simulink model "Commande_2020"  (R2020b)
settings: Solver=FixedStepAuto  StartTime=0.0  StopTime=0.3  FixedStep=1e-6  RelTol=1e-3
libraries: powerlib x37, powerlib_meascontrol x9, spsFuelCellStackLib x4, fuzblock x3, powerlib_extras x2, simulink x1
settings Model: Creator=Abdelhak_Samir  LastModifiedBy=Abdelhak_Samir
settings SolverCC: ZeroCrossAlgorithm=Adaptive
settings DebuggingCC: IgnoredZcDiagnostic=none  UnconnectedInputMsg=none  UnconnectedOutputMsg=none  UnconnectedLineMsg=none
settings ModelReferenceCC: EnableRefExpFcnMdlSchedulingChecks=off
settings RTWCC: GPUComputeCapability=5.0

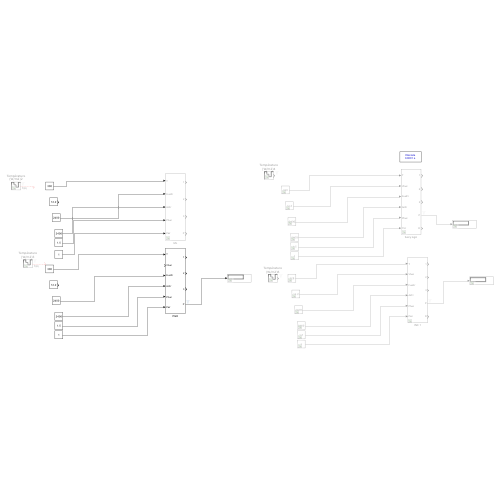
[thumbnail: Simulink's stored preview of the top-level diagram]
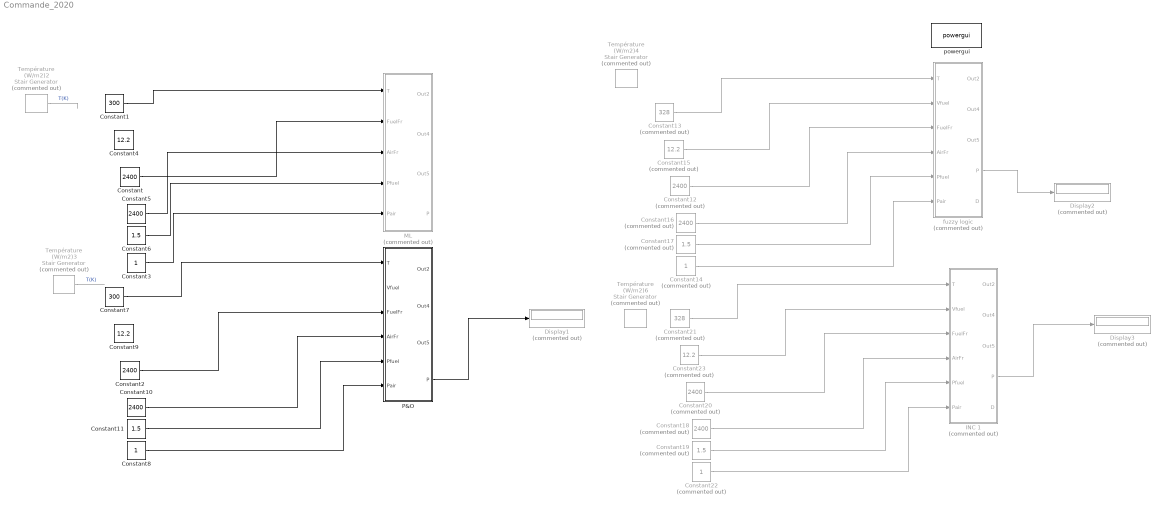
== system Commande_2020 ==
  Constant{,2,5,10} (4 alike) : Constant  Value=2400
  Constant1 : Constant  Value=300
  Constant11 : Constant  Value=1.5
  Constant{12,16,18,20} (4 alike) : Constant  Commented=on  Value=2400
  Constant13 : Constant  Commented=on  Value=328
  Constant14 : Constant  Commented=on
  Constant15 : Constant  Commented=on  Value=12.2
  Constant17 : Constant  Commented=on  Value=1.5
  Constant19 : Constant  Commented=on  Value=1.5
  Constant21 : Constant  Commented=on  Value=328
  Constant22 : Constant  Commented=on
  Constant23 : Constant  Commented=on  Value=12.2
  Constant3 : Constant
  Constant4 : Constant  Value=12.2
  Constant6 : Constant  Value=1.5
  Constant7 : Constant  Value=300
  Constant8 : Constant
  Constant9 : Constant  Value=12.2
  Display1 : Display  Commented=on
  Display2 : Display  Commented=on
  Display3 : Display  Commented=on
  INC 1 : Subsystem  Commented=on
  ML : Subsystem  Commented=on
  P&O : Subsystem
  Température (W/m2){2..4,6} (4 alike) : powerlib_meascontrol/Pulse & Signal Generators/Stair Generator  Commented=on  t=[0, 0.2 , 0.4 , 0.6, 0.8,1]  e=[300,330,320,310,330,330]  Ts=0.00001
  fuzzy logic : Subsystem  Commented=on
  powergui : powerlib/powergui  Priority=1  SimulationMode=Discrete  SampleTime=1e-4  frequency=60  Iterations=50  frequencyindice=0  Pbase=100e6  ErrMax=1e-4  UnitsV=kV  UnitsW=MW  buscounter=0  FunctionMessages=off  echomessages=off  EnableUseOfTLC=off  CurrentSourceSwitches=off  DisableSnubberDevices=off  DisableRonSwitches=off  DisableVfSwitches=off  DisplayEquations=off  AutomaticDiscreteSolvers=off  SolverType=Tustin/Backward Euler (TBE)  Interpol=off  ExternalGateDelay=off  methode=off  Ts=100  x0status=blocks  SPID=on  SwTol=0  HookPort=off  NonlinearTolerance=1e-4  nMaxIteration=100  ContinueOnMaxIteration=off  RestoreLinks=warning  ResistiveCurrentMeasurement=off  Frange=[0:2:500]  Ylog=off  Xlog=on  ShowGrid=off  save=off  variable=ZData  structure=0  ZoomFFT=off  StartTime=0.0  cycles=1  DisplayStyle=1  fundamental=60  FreqAxis=off  MaxFrequency=1000  frequencyindicesteady=1  RmsSteady=1  display=off
  wires:
  Constant8/1 -> P&O/6(Pair)
  Constant10/1 -> P&O/4(AirFr)
  P&O/4(P) -> Display1/1
  Constant11/1 -> P&O/5(Pfuel)
  Constant14/1 -> fuzzy logic/6(Pair)
  Constant12/1 -> fuzzy logic/3(FuelFr)
  Constant15/1 -> fuzzy logic/2(Vfuel)
  Constant16/1 -> fuzzy logic/4(AirFr)
  fuzzy logic/4(P) -> Display2/1
  Constant17/1 -> fuzzy logic/5(Pfuel)
  INC 1/4(P) -> Display3/1
  Constant18/1 -> INC 1/4(AirFr)
  Constant20/1 -> INC 1/3(FuelFr)
  Constant22/1 -> INC 1/6(Pair)
  Constant23/1 -> INC 1/2(Vfuel)
  Constant19/1 -> INC 1/5(Pfuel)
  Constant1/1 -> ML/1(T)
  Constant7/1 -> P&O/1(T)
  Constant13/1 -> fuzzy logic/1(T)
  Constant21/1 -> INC 1/1(T)
  Constant3/1 -> ML/5(Pair)
  Constant6/1 -> ML/4(Pfuel)
  Constant5/1 -> ML/3(AirFr)
  Constant/1 -> ML/2(FuelFr)
  Température (W/m2)2/1 -> ?  "T(K)"
  Température (W/m2)3/1 -> ?  "T(K)"
  Constant2/1 -> P&O/3(FuelFr)

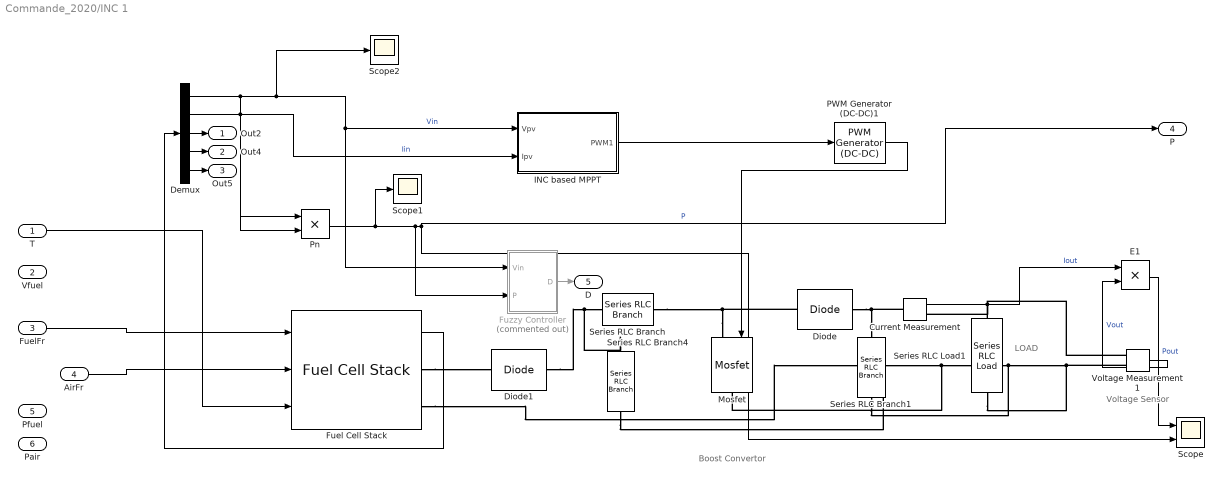
== system Commande_2020/INC 1 ==
  note: LOAD
  note: Boost Convertor
  note: Voltage Sensor
  T : Inport
  Vfuel : Inport  Port=2
  FuelFr : Inport  Port=3
  AirFr : Inport  Port=4
  Pfuel : Inport  Port=5
  Pair : Inport  Port=6
  Current Measurement : powerlib/Measurements/Current Measurement  PhasorSimulation=off  OutputType=Complex  PSBequivalent=0
  Demux : Demux  Outputs=5
  Diode : powerlib/Power Electronics/Diode  Ron=0.001  Lon=0  Vf=0.7  IC=0  UseSnubber=0  Rs=500  Cs=250e-9  Measurements=off
  Diode1 : powerlib/Power Electronics/Diode  Ron=0.001  Lon=0  Vf=0.7  IC=0  UseSnubber=0  Rs=500  Cs=250e-9  Measurements=off
  E1 : Product  Inputs=**
  Fuel Cell Stack : spsFuelCellStackLib/Fuel Cell Stack  PresetModel=No (User-Defined)  FcType=0  Detailed=Detailed  Eoc=[42,35]  NomVI=[52,24.23]  EndVI=[100,20]  Nc=1  n=46  TOp=55  AirFr=2400  SuppPress=[1.5,1]  Comp=[99.95,21,1]  SignX=off  SignY=off  FlowRateH2=on  FlowRateAir=on  SystemTemp=on  SystemPH2=off  SystemPAir=off  FCDyn=off  FC_tau=1  Peak_O2=80  V_Under=10
  Fuzzy Controller : Subsystem  Commented=on
  INC based MPPT : Subsystem
  Mosfet : powerlib/Power Electronics/Mosfet  Ron=0.1  Lon=0  Rd=0.01  Vfd=0.7  IC=0  Rs=1e5  Cs=10^-9  Measurements=off
  PWM Generator (DC-DC)1 : powerlib_meascontrol/Pulse & Signal Generators/PWM Generator (DC-DC)  Fsw=10000  Ts=0
  Pn : Product
  Scope : Scope  NumInputPorts=2
  Scope1 : Scope
  Scope2 : Scope
  Series RLC Branch : powerlib/Elements/Series RLC Branch  LConnTagsString=__new0  RConnTagsString=__new0  BranchType=L  Resistance=1  Inductance=1e-4  SetiL0=off  InitialCurrent=0  Capacitance=1e-6  Setx0=off  InitialVoltage=0  Measurements=None
  Series RLC Branch1 : powerlib/Elements/Series RLC Branch  LConnTagsString=__new0  RConnTagsString=__new0  BranchType=C  Resistance=1  Inductance=1e-4  SetiL0=off  InitialCurrent=0  Capacitance=4700e-6  Setx0=off  InitialVoltage=0  Measurements=None
  Series RLC Branch4 : powerlib/Elements/Series RLC Branch  LConnTagsString=__new0  RConnTagsString=__new0  BranchType=C  Resistance=1  Inductance=1e-4  SetiL0=off  InitialCurrent=0  Capacitance=4700e-5  Setx0=on  InitialVoltage=42  Measurements=None
  Series RLC Load1 : powerlib/Elements/Series RLC Load  LConnTagsString=a  RConnTagsString=__new0  NominalVoltage=50  NominalFrequency=500  ActivePower=33  InductivePower=0  CapacitivePower=0  Setx0=off  InitialVoltage=0  SetiL0=off  InitialCurrent=0  Measurements=None  LoadType=constant Z
  Voltage Measurement1 : powerlib/Measurements/Voltage Measurement  PhasorSimulation=off  OutputType=Complex  PSBequivalent=0
  Out2 : Outport
  Out4 : Outport  Port=2
  Out5 : Outport  Port=3
  P : Outport  Port=4
  D : Outport  Port=5
  wires:
  Current Measurement/1 -> E1/1  "Iout"
  Pn/1 -> P/1, Scope/2, Fuzzy Controller/2(P), Scope1/1  "P"
  PWM Generator (DC-DC)1/1 -> Mosfet/1
  Demux/1 -> Fuzzy Controller/1(Vin), INC based MPPT/1(Vpv), Scope2/1, Pn/1  "Vin"
  Fuzzy Controller/1(D) -> D/1
  Demux/5 -> Out5/1
  Demux/2 -> INC based MPPT/2(Ipv), Pn/2  "Iin"
  FuelFr/1 -> Fuel Cell Stack/1
  Fuel Cell Stack/1 -> Demux/1
  E1/1 -> Scope/1  "Pout"
  AirFr/1 -> Fuel Cell Stack/2
  Voltage Measurement1/1 -> E1/2  "Vout"
  INC based MPPT/1(PWM1) -> PWM Generator (DC-DC)1/1
  Demux/3 -> Out2/1
  Demux/4 -> Out4/1
  T/1 -> Fuel Cell Stack/3
  connections:
  Series RLC Branch4/LConn1 -- Series RLC Branch/LConn1 -- Diode1/RConn1
  Series RLC Branch1/LConn1 -- Diode/RConn1 -- Current Measurement/LConn1
  Fuel Cell Stack/RConn1 -- Diode1/LConn1
  Mosfet/RConn1 -- Fuel Cell Stack/RConn2 -- Series RLC Branch4/RConn1 -- Voltage Measurement1/LConn2 -- Series RLC Load1/RConn1 -- Series RLC Branch1/RConn1
  Current Measurement/RConn1 -- Series RLC Load1/LConn1 -- Voltage Measurement1/LConn1
  Mosfet/LConn1 -- Diode/LConn1 -- Series RLC Branch/RConn1

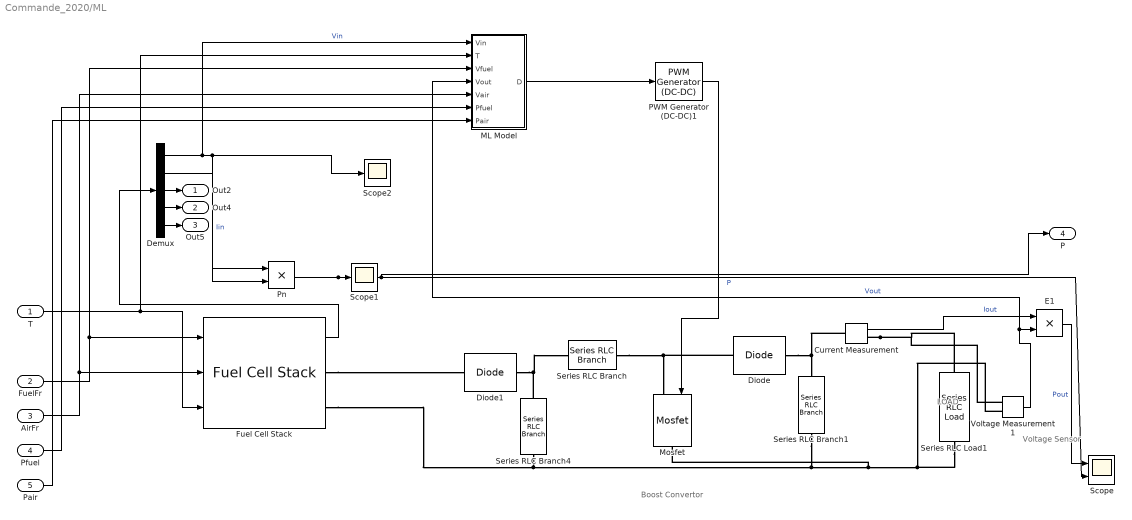
== system Commande_2020/ML ==
  note: LOAD
  note: Voltage Sensor
  note: Boost Convertor
  T : Inport
  FuelFr : Inport  Port=2
  AirFr : Inport  Port=3
  Pfuel : Inport  Port=4
  Pair : Inport  Port=5
  Current Measurement : powerlib/Measurements/Current Measurement  PhasorSimulation=off  OutputType=Complex  PSBequivalent=0
  Demux : Demux  Outputs=5
  Diode : powerlib/Power Electronics/Diode  Ron=0.001  Lon=0  Vf=0.7  IC=0  UseSnubber=0  Rs=500  Cs=250e-9  Measurements=off
  Diode1 : powerlib/Power Electronics/Diode  Ron=0.001  Lon=0  Vf=0.7  IC=0  UseSnubber=0  Rs=500  Cs=250e-9  Measurements=off
  E1 : Product  Inputs=**
  Fuel Cell Stack : spsFuelCellStackLib/Fuel Cell Stack  PresetModel=PEMFC - 1.26 kW - 24 Vdc  FcType=0  Detailed=Detailed  Eoc=[42,35]  NomVI=[52,24.23]  EndVI=[100,20]  Nc=42  n=46  TOp=55  AirFr=2400  SuppPress=[1.5,1]  Comp=[99.95,21,1]  SignX=off  SignY=off  FlowRateH2=on  FlowRateAir=on  SystemTemp=on  SystemPH2=off  SystemPAir=off  FCDyn=off  FC_tau=1  Peak_O2=80  V_Under=10
  ML Model : Subsystem
  Mosfet : powerlib/Power Electronics/Mosfet  Ron=0.1  Lon=0  Rd=0.01  Vfd=0.7  IC=0  Rs=1e5  Cs=10^-9  Measurements=off
  PWM Generator (DC-DC)1 : powerlib_meascontrol/Pulse & Signal Generators/PWM Generator (DC-DC)  Fsw=10000  Ts=0
  Pn : Product
  Scope : Scope  NumInputPorts=2
  Scope1 : Scope
  Scope2 : Scope
  Series RLC Branch : powerlib/Elements/Series RLC Branch  LConnTagsString=__new0  RConnTagsString=__new0  BranchType=L  Resistance=1  Inductance=1e-4  SetiL0=off  InitialCurrent=0  Capacitance=1e-6  Setx0=off  InitialVoltage=0  Measurements=None
  Series RLC Branch1 : powerlib/Elements/Series RLC Branch  LConnTagsString=__new0  RConnTagsString=__new0  BranchType=C  Resistance=1  Inductance=1e-4  SetiL0=off  InitialCurrent=0  Capacitance=4700e-6  Setx0=off  InitialVoltage=0  Measurements=None
  Series RLC Branch4 : powerlib/Elements/Series RLC Branch  LConnTagsString=__new0  RConnTagsString=__new0  BranchType=C  Resistance=1  Inductance=1e-4  SetiL0=off  InitialCurrent=0  Capacitance=4700e-5  Setx0=on  InitialVoltage=42  Measurements=None
  Series RLC Load1 : powerlib/Elements/Series RLC Load  LConnTagsString=a  RConnTagsString=__new0  NominalVoltage=50  NominalFrequency=500  ActivePower=33  InductivePower=0  CapacitivePower=0  Setx0=off  InitialVoltage=0  SetiL0=off  InitialCurrent=0  Measurements=None  LoadType=constant Z
  Voltage Measurement1 : powerlib/Measurements/Voltage Measurement  PhasorSimulation=off  OutputType=Complex  PSBequivalent=0
  Out2 : Outport
  Out4 : Outport  Port=2
  Out5 : Outport  Port=3
  P : Outport  Port=4
  wires:
  Pair/1 -> ML Model/7(Pair)
  FuelFr/1 -> Fuel Cell Stack/1, ML Model/3(Vfuel)
  T/1 -> Fuel Cell Stack/3, ML Model/2(T)
  Fuel Cell Stack/1 -> Demux/1
  Demux/3 -> Out2/1
  Demux/2 -> Pn/2  "Iin"
  Demux/5 -> Out5/1
  E1/1 -> Scope/1  "Pout"
  Pfuel/1 -> ML Model/6(Pfuel)
  Demux/4 -> Out4/1
  Current Measurement/1 -> E1/1  "Iout"
  AirFr/1 -> Fuel Cell Stack/2, ML Model/5(Vair)
  Voltage Measurement1/1 -> ML Model/4(Vout), E1/2  "Vout"
  Pn/1 -> P/1, Scope/2, Scope1/1  "P"
  Demux/1 -> ML Model/1(Vin), Scope2/1, Pn/1  "Vin"
  ML Model/1(D) -> PWM Generator (DC-DC)1/1
  PWM Generator (DC-DC)1/1 -> Mosfet/1
  connections:
  Diode1/RConn1 -- Series RLC Branch4/LConn1 -- Series RLC Branch/LConn1
  Current Measurement/LConn1 -- Series RLC Branch1/LConn1 -- Diode/RConn1
  Series RLC Branch4/RConn1 -- Fuel Cell Stack/RConn2 -- Series RLC Load1/RConn1 -- Voltage Measurement1/LConn2 -- Mosfet/RConn1 -- Series RLC Branch1/RConn1
  Current Measurement/RConn1 -- Series RLC Load1/LConn1 -- Voltage Measurement1/LConn1
  Series RLC Branch/RConn1 -- Diode/LConn1 -- Mosfet/LConn1
  Fuel Cell Stack/RConn1 -- Diode1/LConn1

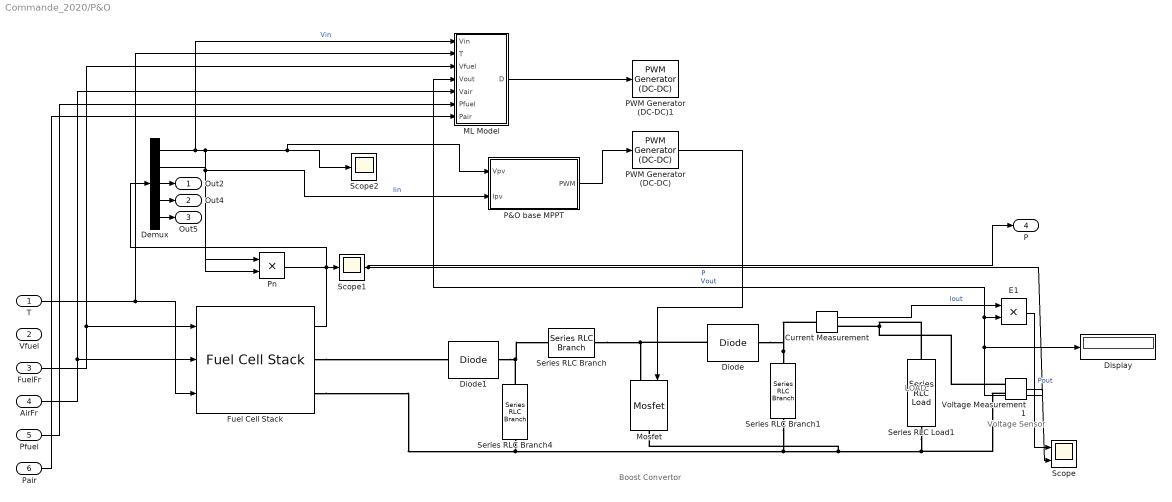
== system Commande_2020/P&O ==
  note: LOAD
  note: Boost Convertor
  note: Voltage Sensor
  T : Inport
  Vfuel : Inport  Port=2
  FuelFr : Inport  Port=3
  AirFr : Inport  Port=4
  Pfuel : Inport  Port=5
  Pair : Inport  Port=6
  Current Measurement : powerlib/Measurements/Current Measurement  PhasorSimulation=off  OutputType=Complex  PSBequivalent=0
  Demux : Demux  Outputs=5
  Diode : powerlib/Power Electronics/Diode  Ron=0.001  Lon=0  Vf=0.7  IC=0  UseSnubber=0  Rs=500  Cs=250e-9  Measurements=off
  Diode1 : powerlib/Power Electronics/Diode  Ron=0.001  Lon=0  Vf=0.7  IC=0  UseSnubber=0  Rs=500  Cs=250e-9  Measurements=off
  Display : Display
  E1 : Product  Inputs=**
  Fuel Cell Stack : spsFuelCellStackLib/Fuel Cell Stack  PresetModel=PEMFC - 1.26 kW - 24 Vdc  FcType=0  Detailed=Detailed  Eoc=[42,35]  NomVI=[52,24.23]  EndVI=[100,20]  Nc=42  n=46  TOp=55  AirFr=2400  SuppPress=[1.5,1]  Comp=[99.95,21,1]  SignX=off  SignY=off  FlowRateH2=on  FlowRateAir=on  SystemTemp=on  SystemPH2=off  SystemPAir=off  FCDyn=off  FC_tau=1  Peak_O2=80  V_Under=10
  ML Model : Subsystem
  Mosfet : powerlib/Power Electronics/Mosfet  Ron=0.1  Lon=0  Rd=0.01  Vfd=0.7  IC=0  Rs=1e5  Cs=10^-9  Measurements=off
  P&O base MPPT : Subsystem
  PWM Generator (DC-DC) : powerlib_meascontrol/Pulse & Signal Generators/PWM Generator (DC-DC)  Fsw=10000  Ts=1e-4
  PWM Generator (DC-DC)1 : powerlib_meascontrol/Pulse & Signal Generators/PWM Generator (DC-DC)  Fsw=10000  Ts=1e-4
  Pn : Product
  Scope : Scope  NumInputPorts=2
  Scope1 : Scope
  Scope2 : Scope
  Series RLC Branch : powerlib/Elements/Series RLC Branch  LConnTagsString=__new0  RConnTagsString=__new0  BranchType=L  Resistance=1  Inductance=1e-4  SetiL0=off  InitialCurrent=0  Capacitance=1e-6  Setx0=off  InitialVoltage=0  Measurements=None
  Series RLC Branch1 : powerlib/Elements/Series RLC Branch  LConnTagsString=__new0  RConnTagsString=__new0  BranchType=C  Resistance=1  Inductance=1e-4  SetiL0=off  InitialCurrent=0  Capacitance=4700e-6  Setx0=off  InitialVoltage=0  Measurements=None
  Series RLC Branch4 : powerlib/Elements/Series RLC Branch  LConnTagsString=__new0  RConnTagsString=__new0  BranchType=C  Resistance=1  Inductance=1e-4  SetiL0=off  InitialCurrent=0  Capacitance=4700e-5  Setx0=on  InitialVoltage=42  Measurements=None
  Series RLC Load1 : powerlib/Elements/Series RLC Load  LConnTagsString=a  RConnTagsString=__new0  NominalVoltage=50  NominalFrequency=500  ActivePower=33  InductivePower=0  CapacitivePower=0  Setx0=off  InitialVoltage=0  SetiL0=off  InitialCurrent=0  Measurements=None  LoadType=constant Z
  Voltage Measurement1 : powerlib/Measurements/Voltage Measurement  PhasorSimulation=off  OutputType=Complex  PSBequivalent=0
  Out2 : Outport
  Out4 : Outport  Port=2
  Out5 : Outport  Port=3
  P : Outport  Port=4
  wires:
  Current Measurement/1 -> E1/1  "Iout"
  Pn/1 -> P/1, Scope/2, Scope1/1  "P"
  Demux/1 -> ML Model/1(Vin), Scope2/1, P&O base MPPT/1(Vpv), Pn/1  "Vin"
  Demux/5 -> Out5/1
  Demux/2 -> P&O base MPPT/2(Ipv), Pn/2  "Iin"
  FuelFr/1 -> Fuel Cell Stack/1, ML Model/3(Vfuel)
  Fuel Cell Stack/1 -> Demux/1
  E1/1 -> Scope/1  "Pout"
  AirFr/1 -> Fuel Cell Stack/2, ML Model/5(Vair)
  Voltage Measurement1/1 -> Display/1, ML Model/4(Vout), E1/2  "Vout"
  Demux/3 -> Out2/1
  Demux/4 -> Out4/1
  T/1 -> ML Model/2(T), Fuel Cell Stack/3
  P&O base MPPT/1(PWM) -> PWM Generator (DC-DC)/1
  ML Model/1(D) -> PWM Generator (DC-DC)1/1
  Pfuel/1 -> ML Model/6(Pfuel)
  Pair/1 -> ML Model/7(Pair)
  PWM Generator (DC-DC)/1 -> Mosfet/1
  connections:
  Series RLC Branch4/LConn1 -- Series RLC Branch/LConn1 -- Diode1/RConn1
  Series RLC Branch1/LConn1 -- Diode/RConn1 -- Current Measurement/LConn1
  Fuel Cell Stack/RConn1 -- Diode1/LConn1
  Fuel Cell Stack/RConn2 -- Voltage Measurement1/LConn2 -- Series RLC Load1/RConn1 -- Mosfet/RConn1 -- Series RLC Branch1/RConn1 -- Series RLC Branch4/RConn1
  Series RLC Load1/LConn1 -- Voltage Measurement1/LConn1 -- Current Measurement/RConn1
  Diode/LConn1 -- Mosfet/LConn1 -- Series RLC Branch/RConn1

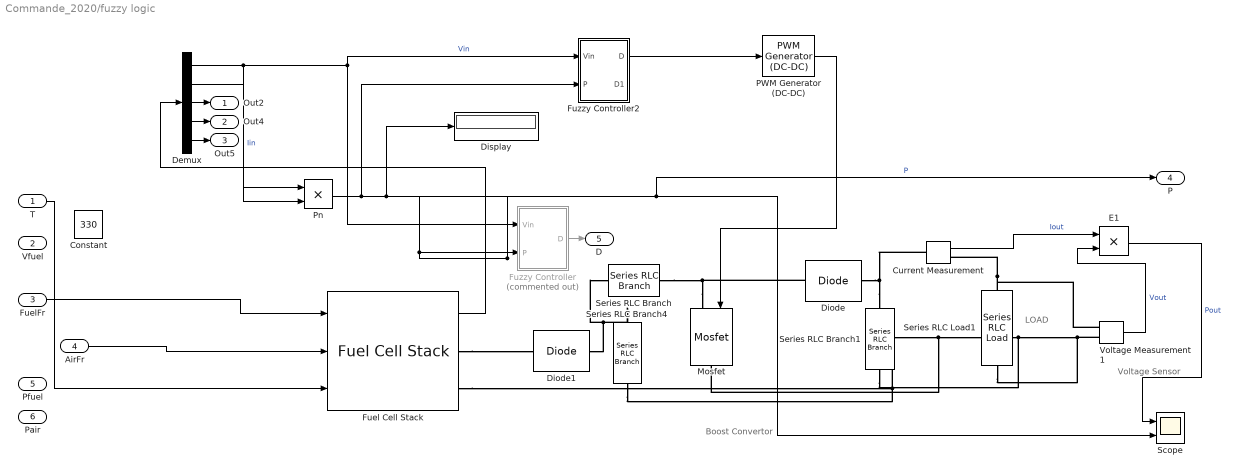
== system Commande_2020/fuzzy logic ==
  note: LOAD
  note: Boost Convertor
  note: Voltage Sensor
  T : Inport
  Vfuel : Inport  Port=2
  FuelFr : Inport  Port=3
  AirFr : Inport  Port=4
  Pfuel : Inport  Port=5
  Pair : Inport  Port=6
  Constant : Constant  Value=330
  Current Measurement : powerlib/Measurements/Current Measurement  PhasorSimulation=off  OutputType=Complex  PSBequivalent=0
  Demux : Demux  Outputs=5
  Diode : powerlib/Power Electronics/Diode  Ron=0.001  Lon=0  Vf=0.7  IC=0  UseSnubber=0  Rs=500  Cs=250e-9  Measurements=off
  Diode1 : powerlib/Power Electronics/Diode  Ron=0.001  Lon=0  Vf=0.7  IC=0  UseSnubber=0  Rs=500  Cs=250e-9  Measurements=off
  Display : Display
  E1 : Product  Inputs=**
  Fuel Cell Stack : spsFuelCellStackLib/Fuel Cell Stack  PresetModel=No (User-Defined)  FcType=0  Detailed=Detailed  Eoc=[42,35]  NomVI=[52,24.23]  EndVI=[100,20]  Nc=1  n=46  TOp=55  AirFr=2400  SuppPress=[1.5,1]  Comp=[99.95,21,1]  SignX=off  SignY=off  FlowRateH2=on  FlowRateAir=on  SystemTemp=on  SystemPH2=off  SystemPAir=off  FCDyn=off  FC_tau=1  Peak_O2=80  V_Under=10
  Fuzzy Controller : Subsystem  Commented=on
  Fuzzy Controller2 : Subsystem
  Mosfet : powerlib/Power Electronics/Mosfet  Ron=0.1  Lon=0  Rd=0.01  Vfd=0.7  IC=0  Rs=1e5  Cs=10^-9  Measurements=off
  PWM Generator (DC-DC) : powerlib_meascontrol/Pulse & Signal Generators/PWM Generator (DC-DC)  Fsw=10000  Ts=0
  Pn : Product
  Scope : Scope  NumInputPorts=2
  Series RLC Branch : powerlib/Elements/Series RLC Branch  LConnTagsString=__new0  RConnTagsString=__new0  BranchType=L  Resistance=1  Inductance=1e-4  SetiL0=off  InitialCurrent=0  Capacitance=1e-6  Setx0=off  InitialVoltage=0  Measurements=None
  Series RLC Branch1 : powerlib/Elements/Series RLC Branch  LConnTagsString=__new0  RConnTagsString=__new0  BranchType=C  Resistance=1  Inductance=1e-4  SetiL0=off  InitialCurrent=0  Capacitance=4700e-6  Setx0=off  InitialVoltage=0  Measurements=None
  Series RLC Branch4 : powerlib/Elements/Series RLC Branch  LConnTagsString=__new0  RConnTagsString=__new0  BranchType=C  Resistance=1  Inductance=1e-4  SetiL0=off  InitialCurrent=0  Capacitance=4700e-5  Setx0=on  InitialVoltage=42  Measurements=None
  Series RLC Load1 : powerlib/Elements/Series RLC Load  LConnTagsString=a  RConnTagsString=__new0  NominalVoltage=50  NominalFrequency=500  ActivePower=33  InductivePower=0  CapacitivePower=0  Setx0=off  InitialVoltage=0  SetiL0=off  InitialCurrent=0  Measurements=None  LoadType=constant Z
  Voltage Measurement1 : powerlib/Measurements/Voltage Measurement  PhasorSimulation=off  OutputType=Complex  PSBequivalent=0
  Out2 : Outport
  Out4 : Outport  Port=2
  Out5 : Outport  Port=3
  P : Outport  Port=4
  D : Outport  Port=5
  wires:
  Current Measurement/1 -> E1/1  "Iout"
  Pn/1 -> Fuzzy Controller2/2(P), Display/1, P/1, Scope/2, Fuzzy Controller/2(P)  "P"
  Demux/1 -> Fuzzy Controller2/1(Vin), Fuzzy Controller/1(Vin), Pn/1  "Vin"
  Fuzzy Controller/1(D) -> D/1
  Demux/5 -> Out5/1
  Demux/2 -> Pn/2  "Iin"
  Fuel Cell Stack/1 -> Demux/1
  E1/1 -> Scope/1  "Pout"
  Voltage Measurement1/1 -> E1/2  "Vout"
  PWM Generator (DC-DC)/1 -> Mosfet/1
  Demux/3 -> Out2/1
  Demux/4 -> Out4/1
  Fuzzy Controller2/1(D) -> PWM Generator (DC-DC)/1
  AirFr/1 -> Fuel Cell Stack/2
  FuelFr/1 -> Fuel Cell Stack/1
  T/1 -> Fuel Cell Stack/3
  connections:
  Series RLC Branch4/LConn1 -- Series RLC Branch/LConn1 -- Diode1/RConn1
  Series RLC Branch1/LConn1 -- Diode/RConn1 -- Current Measurement/LConn1
  Fuel Cell Stack/RConn1 -- Diode1/LConn1
  Mosfet/RConn1 -- Fuel Cell Stack/RConn2 -- Series RLC Branch4/RConn1 -- Series RLC Load1/RConn1 -- Voltage Measurement1/LConn2 -- Series RLC Branch1/RConn1
  Current Measurement/RConn1 -- Voltage Measurement1/LConn1 -- Series RLC Load1/LConn1
  Mosfet/LConn1 -- Diode/LConn1 -- Series RLC Branch/RConn1

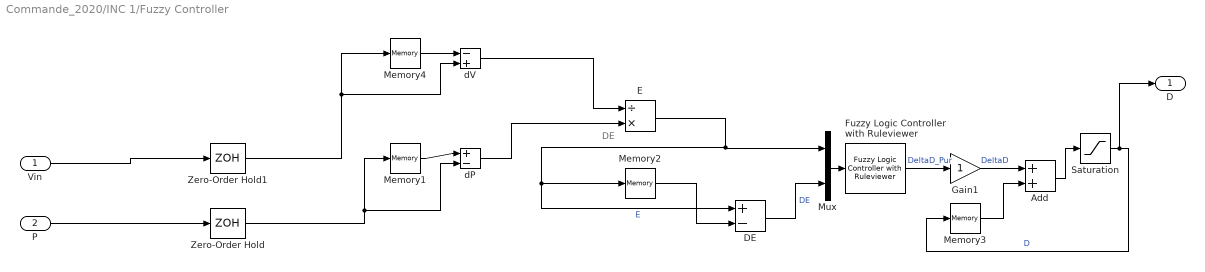
== system Commande_2020/INC 1/Fuzzy Controller ==
  note: DE
  Vin : Inport
  P : Inport  Port=2
  Add : Sum
  DE : Sum  Inputs=+-
  E : Product  Inputs=/*
  Fuzzy Logic Controller with Ruleviewer : fuzblock/Fuzzy Logic  Controller  with Ruleviewer  fismatrix=twnty_five_rules_2  Ts=0.1
  Gain1 : Gain
  Memory1 : Memory  InheritSampleTime=on
  Memory2 : Memory  InheritSampleTime=on
  Memory3 : Memory
  Memory4 : Memory  InheritSampleTime=on
  Mux : Mux  Inputs=2
  Saturation : Saturate  UpperLimit=0.9  LowerLimit=0.1
  Zero-Order Hold : ZeroOrderHold  SampleTime=-1
  Zero-Order Hold1 : ZeroOrderHold  SampleTime=-1
  dP : Sum  Inputs=|+-
  dV : Sum  Inputs=-+
  D : Outport
  wires:
  DE/1 -> Mux/2  "DE"
  Fuzzy Logic Controller with Ruleviewer/1 -> Gain1/1  "DeltaD_Pur"
  Zero-Order Hold/1 -> dP/2, Memory1/1
  dV/1 -> E/1
  dP/1 -> E/2
  E/1 -> DE/1, Memory2/1, Mux/1  "E"
  Mux/1 -> Fuzzy Logic Controller with Ruleviewer/1
  Memory4/1 -> dV/1
  Memory1/1 -> dP/1
  Zero-Order Hold1/1 -> Memory4/1, dV/2
  Gain1/1 -> Add/1  "DeltaD"
  Memory3/1 -> Add/2
  Saturation/1 -> D/1, Memory3/1  "D"
  Memory2/1 -> DE/2
  Add/1 -> Saturation/1
  Vin/1 -> Zero-Order Hold1/1
  P/1 -> Zero-Order Hold/1

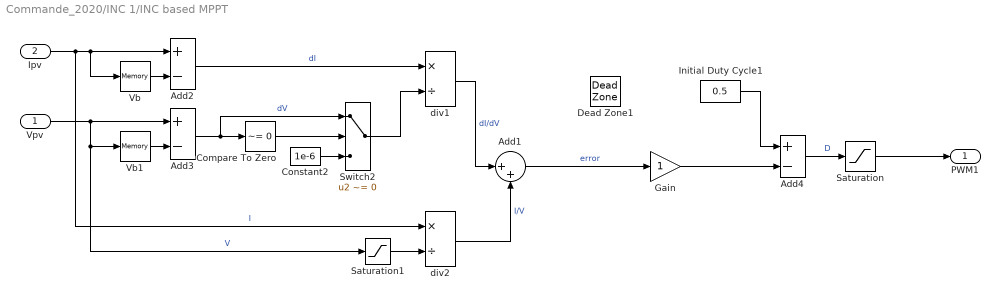
== system Commande_2020/INC 1/INC based MPPT ==
  Vpv : Inport
  Ipv : Inport  Port=2
  Add1 : Sum  Inputs=|++
  Add2 : Sum  Inputs=+-
  Add3 : Sum  Inputs=+-
  Add4 : Sum  Inputs=+-
  Compare To Zero : simulink/Logic and Bit Operations/Compare To Zero  relop=~=  OutDataTypeStr=uint8
  Constant2 : Constant  Value=1e-6
  Dead Zone1 : DeadZone  LowerValue=-0.02  UpperValue=+0.02  SaturateOnIntegerOverflow=on
  Gain : Gain
  Initial Duty Cycle1 : Constant  Value=0.5
  Saturation : Saturate  UpperLimit=0.9  LowerLimit=0.1
  Saturation1 : Saturate  UpperLimit=inf  LowerLimit=eps
  Switch2 : Switch  Criteria=u2 ~= 0
  Vb : Memory  InheritSampleTime=on  LinearizeAsDelay=on
  Vb1 : Memory  InheritSampleTime=on  LinearizeAsDelay=on
  div1 : Product  Inputs=*/  RndMeth=Zero
  div2 : Product  Inputs=*/  RndMeth=Zero
  PWM1 : Outport
  wires:
  Add4/1 -> Saturation/1  "D"
  Gain/1 -> Add4/2
  Initial Duty Cycle1/1 -> Add4/1
  Add3/1 -> Compare To Zero/1, Switch2/1  "dV"
  div2/1 -> Add1/2  "I/V"
  Saturation1/1 -> div2/2
  Vb1/1 -> Add3/2
  Add2/1 -> div1/1  "dI"
  Switch2/1 -> div1/2
  Vb/1 -> Add2/2
  Ipv/1 -> Vb/1, Add2/1, div2/1  "I"
  div1/1 -> Add1/1  "dI/dV"
  Compare To Zero/1 -> Switch2/2
  Constant2/1 -> Switch2/3
  Vpv/1 -> Add3/1, Vb1/1, Saturation1/1  "V"
  Add1/1 -> Gain/1  "error"
  Saturation/1 -> PWM1/1

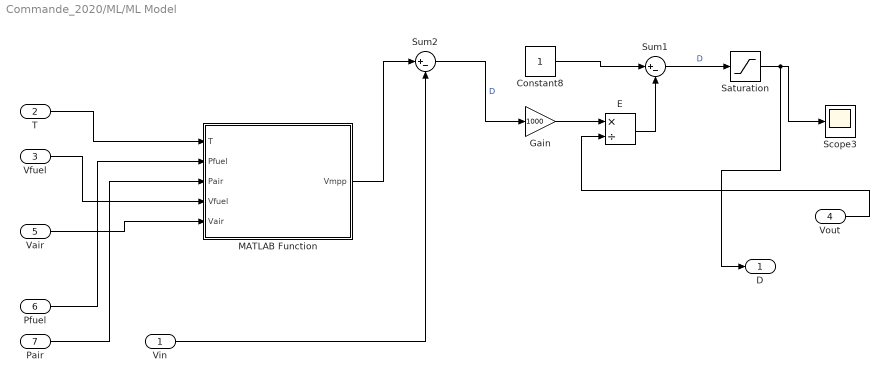
== system Commande_2020/ML/ML Model ==
  Vin : Inport
  T : Inport  Port=2
  Vfuel : Inport  Port=3
  Vout : Inport  Port=4
  Vair : Inport  Port=5
  Pfuel : Inport  Port=6
  Pair : Inport  Port=7
  Constant8 : Constant
  E : Product  Inputs=*/
  Gain : Gain  Gain=1000
  MATLAB Function : MATLAB Function  TreatAsAtomicUnit=on
  Saturation : Saturate  UpperLimit=0.9  LowerLimit=0.1
  Scope3 : Scope
  Sum1 : Sum  Inputs=|+-
  Sum2 : Sum  Inputs=|+-
  D : Outport
  wires:
  Saturation/1 -> D/1, Scope3/1
  Gain/1 -> E/1
  Sum1/1 -> Saturation/1  "D"
  Pair/1 -> MATLAB Function/3(Pair)
  Sum2/1 -> Gain/1  "D"
  E/1 -> Sum1/2
  T/1 -> MATLAB Function/1(T)
  Constant8/1 -> Sum1/1
  Vin/1 -> Sum2/2
  Vout/1 -> E/2
  Pfuel/1 -> MATLAB Function/2(Pfuel)
  Vfuel/1 -> MATLAB Function/4(Vfuel)
  Vair/1 -> MATLAB Function/5(Vair)
  MATLAB Function/1(Vmpp) -> Sum2/1

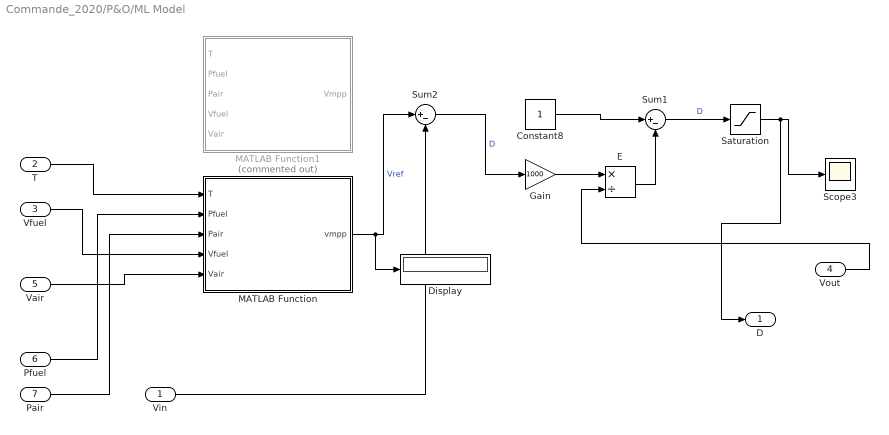
== system Commande_2020/P&O/ML Model ==
  Vin : Inport
  T : Inport  Port=2
  Vfuel : Inport  Port=3
  Vout : Inport  Port=4
  Vair : Inport  Port=5
  Pfuel : Inport  Port=6
  Pair : Inport  Port=7
  Constant8 : Constant
  Display : Display
  E : Product  Inputs=*/
  Gain : Gain  Gain=1000
  MATLAB Function : MATLAB Function  TreatAsAtomicUnit=on
  MATLAB Function1 : MATLAB Function  Commented=on  TreatAsAtomicUnit=on
  Saturation : Saturate  UpperLimit=0.9  LowerLimit=0.1
  Scope3 : Scope
  Sum1 : Sum  Inputs=|+-
  Sum2 : Sum  Inputs=|+-
  D : Outport
  wires:
  Saturation/1 -> D/1, Scope3/1
  Gain/1 -> E/1
  MATLAB Function/1(vmpp) -> Display/1, Sum2/1  "Vref"
  Sum1/1 -> Saturation/1  "D"
  Pair/1 -> MATLAB Function/3(Pair)
  Sum2/1 -> Gain/1  "D"
  E/1 -> Sum1/2
  T/1 -> MATLAB Function/1(T)
  Constant8/1 -> Sum1/1
  Vin/1 -> Sum2/2
  Vout/1 -> E/2
  Pfuel/1 -> MATLAB Function/2(Pfuel)
  Vfuel/1 -> MATLAB Function/4(Vfuel)
  Vair/1 -> MATLAB Function/5(Vair)

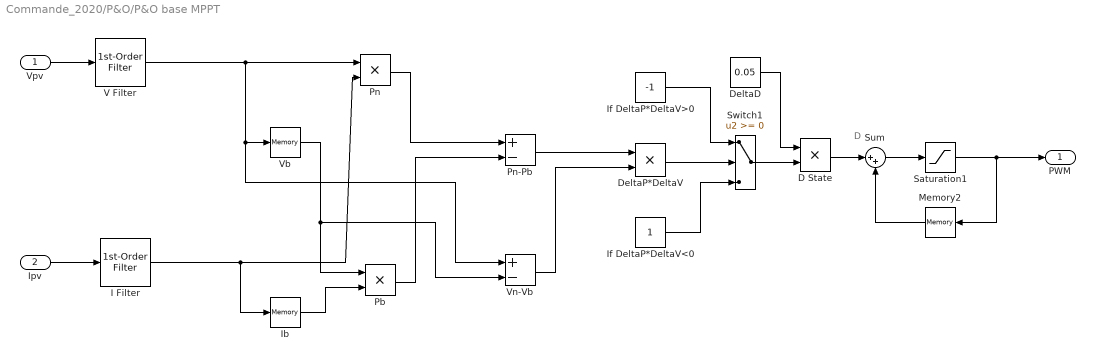
== system Commande_2020/P&O/P&O base MPPT ==
  note: D
  Vpv : Inport
  Ipv : Inport  Port=2
  D State : Product  RndMeth=Zero
  DeltaD : Constant  Value=0.05
  DeltaP*DeltaV : Product  RndMeth=Zero
  I Filter : powerlib_extras/Control  Blocks/1st-Order  Filter  FilterType=Lowpass  Tc=1e-3  Initialize=off  Vac_Init=[0.8 -25 60]  Vdc_Init=-0.4  PlotResponse=off  param1=[1 500 1]
  Ib : Memory  InheritSampleTime=on  LinearizeAsDelay=on
  If DeltaP*DeltaV<0 : Constant
  If DeltaP*DeltaV>0 : Constant  Value=-1
  Memory2 : Memory  InheritSampleTime=on
  Pb : Product  RndMeth=Zero
  Pn : Product  RndMeth=Zero
  Pn-Pb : Sum  Inputs=+-
  Saturation1 : Saturate  UpperLimit=0.9  LowerLimit=0.1
  Sum : Sum  Inputs=|++
  Switch1 : Switch
  V Filter : powerlib_extras/Control  Blocks/1st-Order  Filter  FilterType=Lowpass  Tc=1e-3  Initialize=off  Vac_Init=[0.8 -25 60]  Vdc_Init=-0.4  PlotResponse=off  param1=[1 500 1]
  Vb : Memory  InheritSampleTime=on  LinearizeAsDelay=on
  Vn-Vb : Sum  Inputs=+-
  PWM : Outport
  wires:
  Ipv/1 -> I Filter/1
  If DeltaP*DeltaV<0/1 -> Switch1/3
  Pn/1 -> Pn-Pb/1
  V Filter/1 -> Vn-Vb/1, Vb/1, Pn/1
  Ib/1 -> Pb/2
  DeltaP*DeltaV/1 -> Switch1/2
  Vb/1 -> Vn-Vb/2, Pb/1
  If DeltaP*DeltaV>0/1 -> Switch1/1
  Pn-Pb/1 -> DeltaP*DeltaV/1
  Vn-Vb/1 -> DeltaP*DeltaV/2
  I Filter/1 -> Pn/2, Ib/1
  Vpv/1 -> V Filter/1
  Pb/1 -> Pn-Pb/2
  Switch1/1 -> D State/2
  DeltaD/1 -> D State/1
  D State/1 -> Sum/1
  Sum/1 -> Saturation1/1
  Memory2/1 -> Sum/2
  Saturation1/1 -> PWM/1, Memory2/1

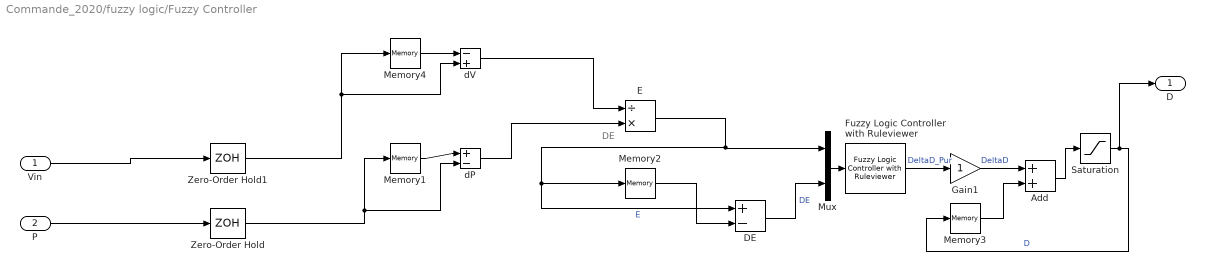
== system Commande_2020/fuzzy logic/Fuzzy Controller ==
  note: DE
  Vin : Inport
  P : Inport  Port=2
  Add : Sum
  DE : Sum  Inputs=+-
  E : Product  Inputs=/*
  Fuzzy Logic Controller with Ruleviewer : fuzblock/Fuzzy Logic  Controller  with Ruleviewer  fismatrix=twnty_five_rules_2  Ts=0.1
  Gain1 : Gain
  Memory1 : Memory  InheritSampleTime=on
  Memory2 : Memory  InheritSampleTime=on
  Memory3 : Memory
  Memory4 : Memory  InheritSampleTime=on
  Mux : Mux  Inputs=2
  Saturation : Saturate  UpperLimit=0.9  LowerLimit=0.1
  Zero-Order Hold : ZeroOrderHold  SampleTime=-1
  Zero-Order Hold1 : ZeroOrderHold  SampleTime=-1
  dP : Sum  Inputs=|+-
  dV : Sum  Inputs=-+
  D : Outport
  wires:
  DE/1 -> Mux/2  "DE"
  Fuzzy Logic Controller with Ruleviewer/1 -> Gain1/1  "DeltaD_Pur"
  Zero-Order Hold/1 -> dP/2, Memory1/1
  dV/1 -> E/1
  dP/1 -> E/2
  E/1 -> DE/1, Memory2/1, Mux/1  "E"
  Mux/1 -> Fuzzy Logic Controller with Ruleviewer/1
  Memory4/1 -> dV/1
  Memory1/1 -> dP/1
  Zero-Order Hold1/1 -> Memory4/1, dV/2
  Gain1/1 -> Add/1  "DeltaD"
  Memory3/1 -> Add/2
  Saturation/1 -> D/1, Memory3/1  "D"
  Memory2/1 -> DE/2
  Add/1 -> Saturation/1
  Vin/1 -> Zero-Order Hold1/1
  P/1 -> Zero-Order Hold/1

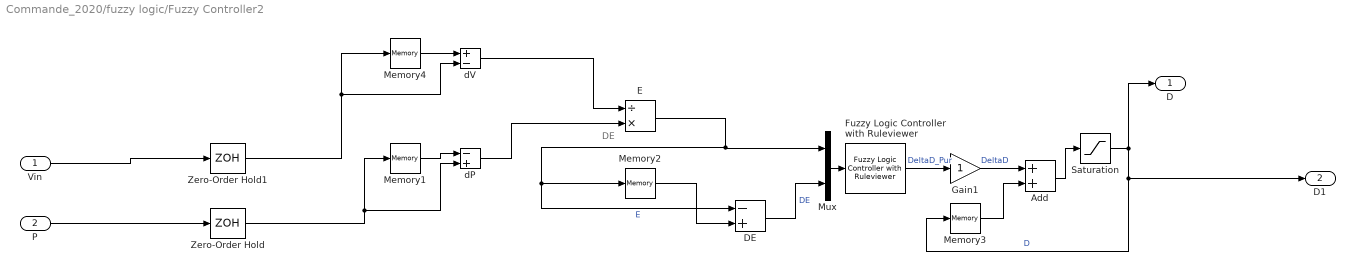
== system Commande_2020/fuzzy logic/Fuzzy Controller2 ==
  note: DE
  Vin : Inport
  P : Inport  Port=2
  Add : Sum
  DE : Sum  Inputs=-+
  E : Product  Inputs=/*
  Fuzzy Logic Controller with Ruleviewer : fuzblock/Fuzzy Logic  Controller  with Ruleviewer  fismatrix=twnty_five_rules_5  Ts=1
  Gain1 : Gain
  Memory1 : Memory  InheritSampleTime=on
  Memory2 : Memory  InheritSampleTime=on
  Memory3 : Memory
  Memory4 : Memory  InheritSampleTime=on
  Mux : Mux  Inputs=2
  Saturation : Saturate  UpperLimit=0.9  LowerLimit=0.1
  Zero-Order Hold : ZeroOrderHold  SampleTime=-1
  Zero-Order Hold1 : ZeroOrderHold  SampleTime=-1
  dP : Sum  Inputs=-+
  dV : Sum  Inputs=+-
  D : Outport
  D1 : Outport  Port=2
  wires:
  DE/1 -> Mux/2  "DE"
  Fuzzy Logic Controller with Ruleviewer/1 -> Gain1/1  "DeltaD_Pur"
  Zero-Order Hold/1 -> dP/2, Memory1/1
  dV/1 -> E/1
  dP/1 -> E/2
  E/1 -> DE/1, Memory2/1, Mux/1  "E"
  Mux/1 -> Fuzzy Logic Controller with Ruleviewer/1
  Memory4/1 -> dV/1
  Memory1/1 -> dP/1
  Zero-Order Hold1/1 -> Memory4/1, dV/2
  Gain1/1 -> Add/1  "DeltaD"
  Memory3/1 -> Add/2
  Saturation/1 -> D/1, D1/1, Memory3/1  "D"
  Memory2/1 -> DE/2
  Add/1 -> Saturation/1
  Vin/1 -> Zero-Order Hold1/1
  P/1 -> Zero-Order Hold/1

== matlab function Commande_2020/P&O/ML Model/MATLAB Function ==
  data: T input; vmpp output; Pfuel input; Pair input; Vfuel input; Vair input
function vmpp = fcn(T, Pfuel, Pair, Vfuel, Vair)
    vmpp = predict_vmpp(T, Pfuel, Pair, Vfuel, Vair);
end

== matlab function Commande_2020/ML/ML Model/MATLAB Function ==
  data: T input; Vmpp output; Pfuel input; Pair input; Vfuel input; Vair input
function Vmpp = fcn(T, Pfuel, Pair, Vfuel, Vair)

    Vmpp = 0.0; % Predefine output as double to satisfy Simulink
    Vmpp = load_pytorch_model(T, Pfuel, Pair, Vfuel, Vair);
end

== matlab function Commande_2020/P&O/ML Model/MATLAB Function1 ==
  data: T input; Vmpp output; Pfuel input; Pair input; Vfuel input; Vair input
function Vmpp = fcn(T, Pfuel, Pair, Vfuel, Vair)

    Vmpp = 0.0; % Predefine output as double to satisfy Simulink
    Vmpp = load_pytorch_model(T, Pfuel, Pair, Vfuel, Vair);
end
